simulink model "plant_literature"  (R2024a)
settings: Solver=FixedStepAuto  StartTime=0.0  StopTime=10  FixedStep=0.005
model mask{considerFem1=1, considerFem2=1, considerFg=1}
  mask prompts: considerFem1 "Upper inductance"; considerFem2 "Lower inductance"; considerFg "Gravity"
InitFcn:
  | run("initial_conditions.m")
  | load("parameters_literature.mat")
model workspace (MAT data in the model file):
  considerFem1 = 1
  considerFem2 = 1
  considerFg = 1
values from neighbouring files (symbols this model uses):
  ci = -0.4    [init.m]    (also in maglev_init.m = 0.0243)
  fiP1 = 1.4142 * 1e-4    (= 0.00014142)    [init.m]    (also in maglev_init.m)
  fiP2 = 4.5626 *1e-3    (= 0.0045626)    [init.m]    (also in maglev_init.m)
  g = 9.81    [init.m]    (also in maglev_init.m)
  H = 98.00 * 1e-3    (= 0.098)    [maglev_init.m]
  ki = 4.4    [init.m]    (also in maglev_init.m = 2.5165)
  m = 0.06157    [init.m]
  r = 30 * 1e-3    (= 0.03)    [init.m]    (also in maglev_init.m = 0.030625)
undefined symbols (not defined in the file or in its folder): FemP1, FemP2, v0, x_eq, z0
settings Model: ExtModeArchiveFileName=test  ExtModeArchiveDirName=C:\Users\Bocchio\OneDrive\University\Lab - Mechatronics\MagLev\results\realtime  ParameterArgumentNames=considerFem1,considerFem2,considerFg  Creator=User  LastModifiedBy=Bocchio
settings SolverCC: ZeroCrossAlgorithm=Adaptive
settings DataIOCC: SaveFormat=Array  SaveOutput=off  SignalLogging=off  SaveTime=off
settings DebuggingCC: IgnoredZcDiagnostic=none  UnconnectedInputMsg=warning  UnconnectedOutputMsg=warning  UnconnectedLineMsg=warning
settings HardwareCC: ProdBitPerPointer=32  ProdBitPerSizeT=32  ProdBitPerPtrDiffT=32  ProdLargestAtomicFloat=None  ProdEndianess=Unspecified  ProdWordSize=32  ProdHWDeviceType=Custom Processor->Custom Processor
settings ModelReferenceCC: EnableRefExpFcnMdlSchedulingChecks=on
settings RTWCC: Description=MLS2EM-RTDAC/USB2 (Visual C/C++)  SystemTargetFile=mls2em_rtcon_usb2.tlc  TemplateMakefile=MLS2EM_RTCON_VC_USB2_x64.tmf  GPUComputeCapability=3.5  DLArmComputeVersion=19.05
settings STFCustomTargetCC: ModelReferenceCompliant=off  CombineOutputUpdateFcns=on  MatFileLogging=on  GRTInterface=off  UseToolchainInfoCompliant=off  SystemTargetFile=mls2em_rtcon_usb2.tlc
settings GRTTargetCC: ModelReferenceCompliant=off  ParMdlRefBuildCompliant=off  CompOptLevelCompliant=off  ConcurrentExecutionCompliant=off  CPPClassGenCompliant=off  UseToolchainInfoCompliant=off  ExtMode=on  ExtModeMexFile=rtcon_ext_comm

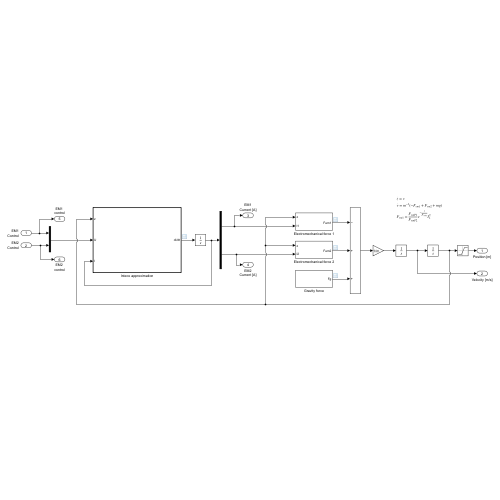
[thumbnail: Simulink's stored preview of the top-level diagram]
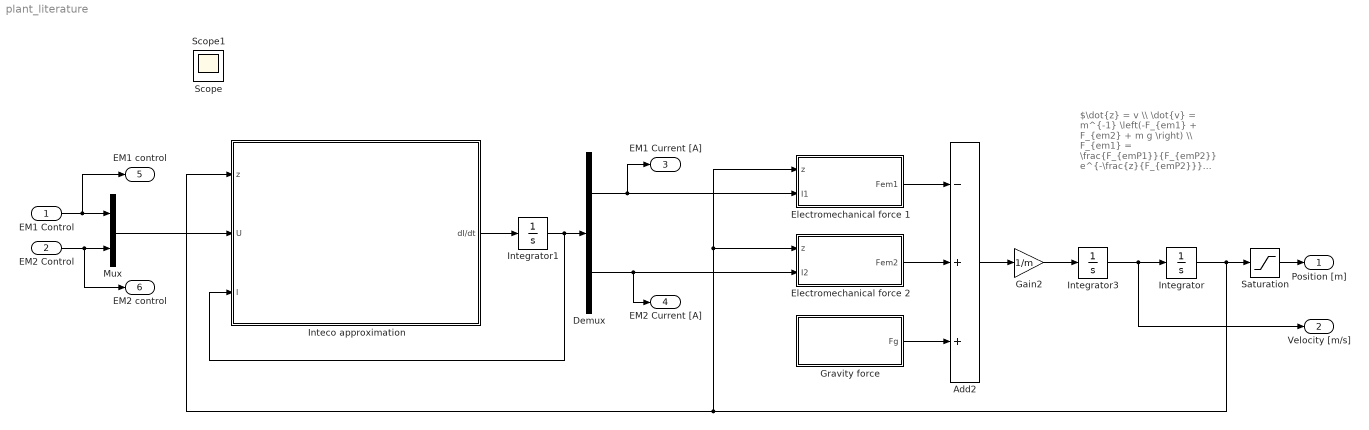
== system plant_literature ==
  note: $\dot{z} = v \\ \dot{v} = m^{-1} \left(-F_{em1} + F_{em2} + m g \right) \\ F_{em1} = \frac{F_{emP1}}{F_{emP2}} e^{-\frac{z}{F_{emP2}}} I_1^2$
  EM1 Control : Inport
  EM2 Control : Inport  Port=2
  Add2 : Sum  Inputs=-++
  Demux : Demux  Outputs=2
  Electromechanical force 1 : Subsystem
  Electromechanical force 2 : Subsystem
  Gain2 : Gain  Gain=1/m
  Gravity force : Subsystem
  Inteco approximation : Subsystem  TreatAsAtomicUnit=on  VariantControl=currentDynamicModel==1
  Integrator : Integrator  InitialCondition=z0
  Integrator1 : Integrator  InitialCondition=x_eq(3:4)
  Integrator3 : Integrator  InitialCondition=v0
  Mux : Mux  Inputs=2
  Saturation : Saturate  UpperLimit=H - 2*r  LowerLimit=0
  Position [m] : Outport
  Velocity [m/s] : Outport  Port=2
  EM1 Current [A] : Outport  Port=3
  EM2 Current [A] : Outport  Port=4
  EM1 control : Outport  Port=5
  EM2 control : Outport  Port=6
  Scope : Scope
  Scope1 : Scope
  wires:
  Integrator3/1 -> Velocity [m/s]/1, Integrator/1
  Electromechanical force 2/1(Fem2) -> Add2/2
  Add2/1 -> Gain2/1
  Mux/1 -> Inteco approximation/2(U)
  Integrator1/1 -> Inteco approximation/3(I), Demux/1
  Inteco approximation/1(dI/dt) -> Integrator1/1
  Gain2/1 -> Integrator3/1
  Electromechanical force 1/1(Fem1) -> Add2/1
  Saturation/1 -> Position [m]/1
  EM2 Control/1 -> EM2 control/1, Mux/2
  Demux/2 -> EM2 Current [A]/1, Electromechanical force 2/2(I2)
  Demux/1 -> EM1 Current [A]/1, Electromechanical force 1/2(I1)
  Gravity force/1(Fg) -> Add2/3
  EM1 Control/1 -> EM1 control/1, Mux/1
  Integrator/1 -> Saturation/1, Inteco approximation/1(z), Electromechanical force 1/1(z), Electromechanical force 2/1(z)

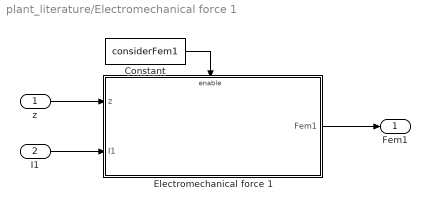
== system plant_literature/Electromechanical force 1 ==
  z : Inport
  I1 : Inport  Port=2
  Constant : Constant  Value=considerFem1
  Electromechanical force 1 : Subsystem  TreatAsAtomicUnit=on
  Fem1 : Outport
  wires:
  z/1 -> Electromechanical force 1/1(z)
  Electromechanical force 1/1(Fem1) -> Fem1/1
  Constant/1 -> Electromechanical force 1/Enable
  I1/1 -> Electromechanical force 1/2(I1)

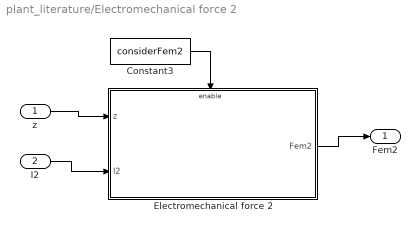
== system plant_literature/Electromechanical force 2 ==
  z : Inport
  I2 : Inport  Port=2
  Constant3 : Constant  Value=considerFem2
  Electromechanical force 2 : Subsystem  TreatAsAtomicUnit=on
  Fem2 : Outport
  wires:
  Constant3/1 -> Electromechanical force 2/Enable
  Electromechanical force 2/1(Fem2) -> Fem2/1
  z/1 -> Electromechanical force 2/1(z)
  I2/1 -> Electromechanical force 2/2(I2)

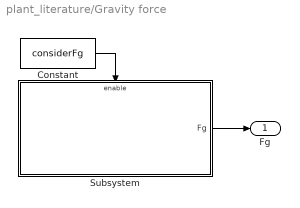
== system plant_literature/Gravity force ==
  Constant : Constant  Value=considerFg
  Subsystem : Subsystem
  Fg : Outport
  wires:
  Subsystem/1(Fg) -> Fg/1
  Constant/1 -> Subsystem/Enable

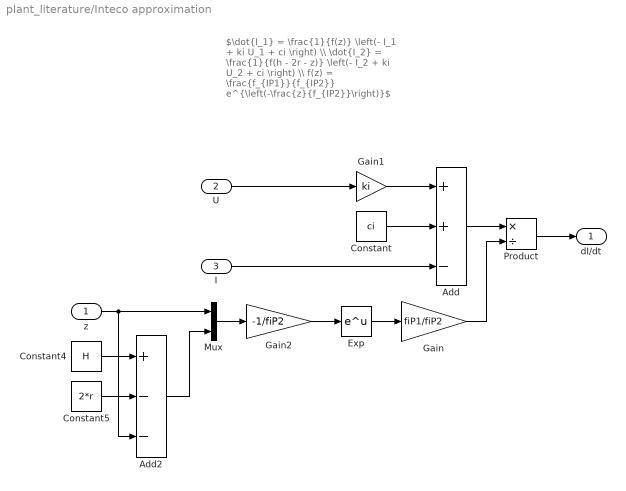
== system plant_literature/Inteco approximation ==
  note: $\dot{I_1} = \frac{1}{f(z)} \left(- I_1 + ki U_1 + ci \right) \\ \dot{I_2} = \frac{1}{f(h - 2r - z)} \left(- I_2 + ki U_2 + ci \right) \\ f(z) = \frac{f_{IP1}}{f_{IP2}} e^{\left(-\frac{z}{f_{IP2}}\right)}$
  z : Inport
  U : Inport  Port=2
  I : Inport  Port=3
  Add : Sum  Inputs=++-
  Add2 : Sum  Inputs=+--
  Constant : Constant  Value=ci
  Constant4 : Constant  Value=H
  Constant5 : Constant  Value=2*r
  Exp : Math
  Gain : Gain  Gain=fiP1/fiP2
  Gain1 : Gain  Gain=ki
  Gain2 : Gain  Gain=-1/fiP2
  Mux : Mux  Inputs=2
  Product : Product  Inputs=*/
  dI/dt : Outport
  wires:
  Exp/1 -> Gain/1
  I/1 -> Add/3
  Gain2/1 -> Exp/1
  U/1 -> Gain1/1
  Constant/1 -> Add/2
  Gain1/1 -> Add/1
  Add/1 -> Product/1
  Gain/1 -> Product/2
  Product/1 -> dI/dt/1
  Mux/1 -> Gain2/1
  Add2/1 -> Mux/2
  Constant5/1 -> Add2/2
  Constant4/1 -> Add2/1
  z/1 -> Add2/3, Mux/1

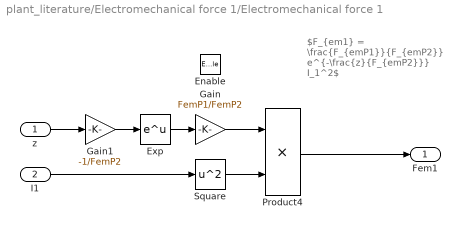
== system plant_literature/Electromechanical force 1/Electromechanical force 1 ==
  note: $F_{em1} = \frac{F_{emP1}}{F_{emP2}} e^{-\frac{z}{F_{emP2}}} I_1^2$
  z : Inport
  I1 : Inport  Port=2
  Enable : EnablePort
  Exp : Math
  Gain : Gain  Gain=FemP1/FemP2
  Gain1 : Gain  Gain=-1/FemP2
  Product4 : Product
  Square : Math  Operator=square
  Fem1 : Outport
  wires:
  I1/1 -> Square/1
  Gain/1 -> Product4/1
  Product4/1 -> Fem1/1
  z/1 -> Gain1/1
  Square/1 -> Product4/2
  Exp/1 -> Gain/1
  Gain1/1 -> Exp/1

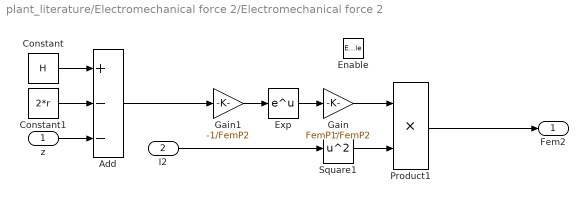
== system plant_literature/Electromechanical force 2/Electromechanical force 2 ==
  z : Inport
  I2 : Inport  Port=2
  Enable : EnablePort
  Add : Sum  Inputs=+--
  Constant : Constant  Value=H
  Constant1 : Constant  Value=2*r
  Exp : Math
  Gain : Gain  Gain=FemP1/FemP2
  Gain1 : Gain  Gain=-1/FemP2
  Product1 : Product
  Square1 : Math  Operator=square
  Fem2 : Outport  OutputWhenDisabled=reset  InitialOutput=0
  wires:
  Product1/1 -> Fem2/1
  Gain/1 -> Product1/1
  I2/1 -> Square1/1
  z/1 -> Add/3
  Square1/1 -> Product1/2
  Gain1/1 -> Exp/1
  Exp/1 -> Gain/1
  Add/1 -> Gain1/1
  Constant1/1 -> Add/2
  Constant/1 -> Add/1

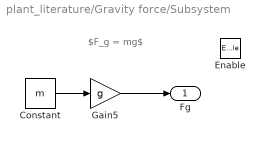
== system plant_literature/Gravity force/Subsystem ==
  note: $F_g = mg$
  Enable : EnablePort
  Constant : Constant  Value=m
  Gain5 : Gain  Gain=g
  Fg : Outport
  wires:
  Gain5/1 -> Fg/1
  Constant/1 -> Gain5/1
